simulink model "Moorer"  (R2023a)
settings: Solver=VariableStepAuto  StartTime=0.0  StopTime=5  RelTol=1e-3
settings Model: Creator=86198  LastModifiedBy=86198

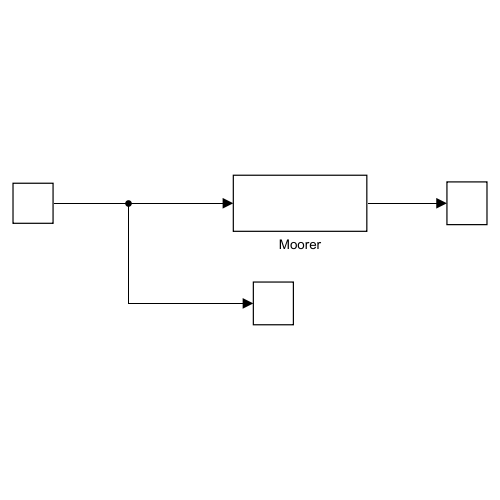
[thumbnail: Simulink's stored preview of the top-level diagram]
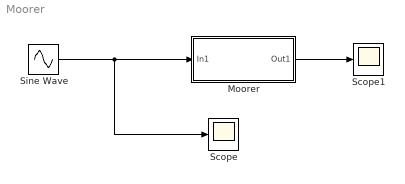
== system Moorer ==
  Moorer : Subsystem
  Scope : Scope
  Scope1 : Scope
  Sine Wave : Sin  Frequency=2*pi*1125  SampleTime=1/48000
  wires:
  Moorer/1(Out1) -> Scope1/1
  Sine Wave/1 -> Moorer/1(In1), Scope/1

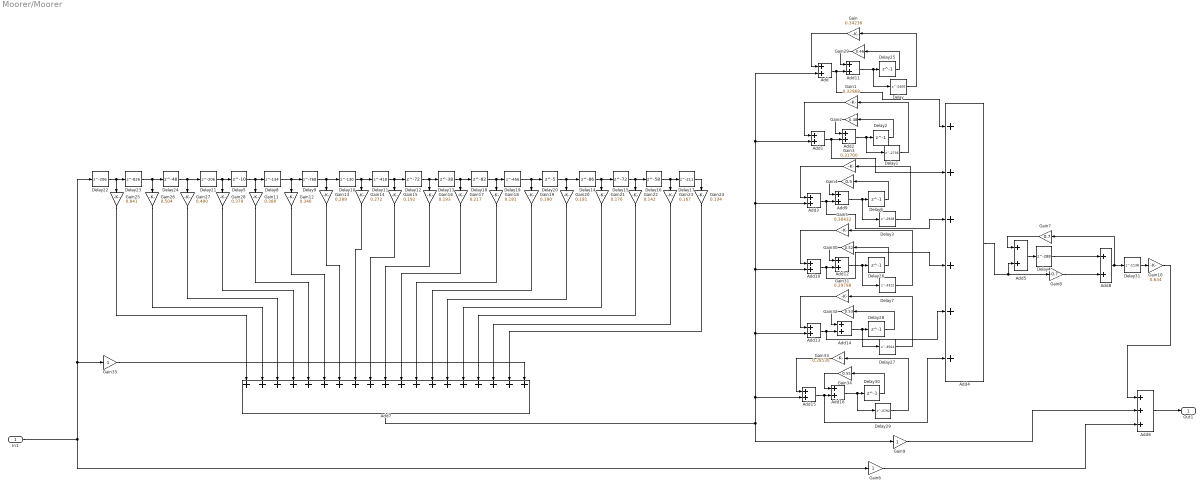
== system Moorer/Moorer ==
  In1 : Inport
  Add{,1..3,5,8..16} (14 alike) : Sum
  Add4 : Sum  Inputs=++++++
  Add6 : Sum  Inputs=+++
  Add7 : Sum  Inputs=+++++++++++++++++++
  Delay : Delay  DelayLength=2400
  Delay1 : Delay  DelayLength=2736
  Delay10 : Delay  DelayLength=130
  Delay11 : Delay  DelayLength=418
  Delay12 : Delay  DelayLength=72
  Delay13 : Delay  DelayLength=38
  Delay14 : Delay  DelayLength=86
  Delay15 : Delay  DelayLength=72
  Delay16 : Delay  DelayLength=58
  Delay17 : Delay  DelayLength=211
  Delay18 : Delay  DelayLength=82
  Delay19 : Delay  DelayLength=456
  Delay{2,6,25..26,28,30} (6 alike) : Delay  DelayLength=1
  Delay20 : Delay  DelayLength=5
  Delay21 : Delay  DelayLength=206
  Delay22 : Delay  DelayLength=206
  Delay23 : Delay  DelayLength=826
  Delay24 : Delay  DelayLength=48
  Delay27 : Delay  DelayLength=3504
  Delay29 : Delay  DelayLength=3792
  Delay3 : Delay  DelayLength=2928
  Delay31 : Delay  DelayLength=1138
  Delay4 : Delay  DelayLength=288
  Delay5 : Delay  DelayLength=10
  Delay7 : Delay  DelayLength=3312
  Delay8 : Delay  DelayLength=134
  Delay9 : Delay  DelayLength=768
  Gain : Gain  Gain=0.34236
  Gain1 : Gain  Gain=0.32968
  Gain10 : Gain  Gain=0.634
  Gain11 : Gain  Gain=0.380
  Gain12 : Gain  Gain=0.346
  Gain13 : Gain  Gain=0.289
  Gain14 : Gain  Gain=0.272
  Gain15 : Gain  Gain=0.192
  Gain16 : Gain  Gain=0.193
  Gain17 : Gain  Gain=0.217
  Gain18 : Gain  Gain=0.181
  Gain19 : Gain  Gain=0.180
  Gain2 : Gain  Gain=0.48
  Gain20 : Gain  Gain=0.181
  Gain21 : Gain  Gain=0.176
  Gain22 : Gain  Gain=0.142
  Gain23 : Gain  Gain=0.167
  Gain24 : Gain  Gain=0.134
  Gain25 : Gain  Gain=0.841
  Gain26 : Gain  Gain=0.504
  Gain27 : Gain  Gain=0.490
  Gain28 : Gain  Gain=0.379
  Gain29 : Gain  Gain=0.46
  Gain3 : Gain  Gain=0.31700
  Gain30 : Gain  Gain=0.52
  Gain31 : Gain  Gain=0.29798
  Gain32 : Gain  Gain=0.53
  Gain33 : Gain  Gain=0.28530
  Gain34 : Gain  Gain=0.55
  Gain35 : Gain
  Gain4 : Gain  Gain=0.5
  Gain5 : Gain  Gain=0.30432
  Gain6 : Gain
  Gain7 : Gain  Gain=0.7
  Gain8 : Gain  Gain=-0.7
  Gain9 : Gain
  Out1 : Outport
  wires:
  Gain/1 -> Add/1
  Add4/1 -> Add5/2, Gain8/1
  Delay4/1 -> Add8/1
  Gain7/1 -> Add5/1
  Add8/1 -> Delay31/1, Gain7/1
  Add6/1 -> Out1/1
  Gain10/1 -> Add6/1
  Gain8/1 -> Add8/2
  In1/1 -> Gain6/1, Delay22/1, Gain35/1
  Add7/1 -> Add15/2, Add13/2, Add10/2, Add3/2, Add/2, Add1/2, Gain9/1
  Delay5/1 -> Delay8/1, Gain11/1
  Delay8/1 -> Delay9/1, Gain12/1
  Delay9/1 -> Delay10/1, Gain13/1
  Delay10/1 -> Delay11/1, Gain14/1
  Delay11/1 -> Delay12/1, Gain15/1
  Delay12/1 -> Delay13/1, Gain16/1
  Delay13/1 -> Delay18/1, Gain17/1
  Delay14/1 -> Delay15/1, Gain21/1
  Delay19/1 -> Delay20/1, Gain19/1
  Delay20/1 -> Delay14/1, Gain20/1
  Delay18/1 -> Delay19/1, Gain18/1
  Delay15/1 -> Delay16/1, Gain22/1
  Delay16/1 -> Delay17/1, Gain23/1
  Delay17/1 -> Gain24/1
  Delay21/1 -> Delay5/1, Gain28/1
  Delay23/1 -> Delay24/1, Gain26/1
  Delay24/1 -> Delay21/1, Gain27/1
  Delay22/1 -> Delay23/1, Gain25/1
  Gain25/1 -> Add7/1
  Gain26/1 -> Add7/2
  Gain27/1 -> Add7/3
  Gain28/1 -> Add7/4
  Gain11/1 -> Add7/5
  Gain12/1 -> Add7/6
  Gain13/1 -> Add7/7
  Gain14/1 -> Add7/8
  Gain15/1 -> Add7/9
  Gain16/1 -> Add7/10
  Gain17/1 -> Add7/11
  Gain18/1 -> Add7/12
  Gain19/1 -> Add7/13
  Gain20/1 -> Add7/14
  Gain21/1 -> Add7/15
  Gain22/1 -> Add7/16
  Gain23/1 -> Add7/17
  Gain24/1 -> Add7/18
  Add5/1 -> Delay4/1
  Add/1 -> Add4/1, Add11/2
  Add11/1 -> Delay/1, Delay25/1
  Delay25/1 -> Gain29/1
  Gain29/1 -> Add11/1
  Add2/1 -> Delay1/1, Delay2/1
  Delay2/1 -> Gain2/1
  Gain1/1 -> Add1/1
  Add1/1 -> Add4/2, Add2/2
  Gain2/1 -> Add2/1
  Add9/1 -> Delay3/1, Delay6/1
  Delay6/1 -> Gain4/1
  Delay3/1 -> Gain3/1
  Gain3/1 -> Add3/1
  Add3/1 -> Add4/3, Add9/2
  Gain4/1 -> Add9/1
  Add12/1 -> Delay7/1, Delay26/1
  Delay26/1 -> Gain30/1
  Delay7/1 -> Gain5/1
  Gain5/1 -> Add10/1
  Add10/1 -> Add4/4, Add12/2
  Gain30/1 -> Add12/1
  Add14/1 -> Delay27/1, Delay28/1
  Delay28/1 -> Gain32/1
  Delay27/1 -> Gain31/1
  Gain31/1 -> Add13/1
  Add13/1 -> Add4/5, Add14/2
  Gain32/1 -> Add14/1
  Add16/1 -> Delay29/1, Delay30/1
  Delay30/1 -> Gain34/1
  Delay29/1 -> Gain33/1
  Gain33/1 -> Add15/1
  Add15/1 -> Add4/6, Add16/2
  Gain34/1 -> Add16/1
  Delay1/1 -> Gain1/1
  Delay/1 -> Gain/1
  Delay31/1 -> Gain10/1
  Gain35/1 -> Add7/19
  Gain9/1 -> Add6/2
  Gain6/1 -> Add6/3
